simulink model "ADCS_FP5_RJF_Linear"  (R2024b)
settings: Solver=VariableStepAuto  StartTime=0.0  StopTime=tspan  FixedStep=10  RelTol=1e-4
values from neighbouring files (symbols this model uses):
  E_b_ECI_0 = rotm2eul(C_b_ECI_0)    [AERO421_FP5_RJF.m]
  J = diag([1200,2000,2800])    [AERO421_FP5_RJF.m]
  K = -15    [AERO421_FP5_RJF.m]
  q_b_ECI_0 = -rotm2quat(C_b_ECI_0)    [AERO421_FP5_RJF.m]
  T = [0;0;0]    [AERO421_FP5_RJF.m]
  w_b_ECI_0 = [-0.05; 0.03; 0.2]    [AERO421_FP5_RJF.m]
undefined symbols (not defined in the file or in its folder): Kd, Kp
settings Model: Creator=emehiel  LastModifiedBy=rosha
settings SolverCC: AlgebraicLoopSolver=TrustRegion
settings DebuggingCC: UnconnectedInputMsg=warning  UnconnectedOutputMsg=warning  UnconnectedLineMsg=warning
settings ModelReferenceCC: EnableRefExpFcnMdlSchedulingChecks=on
settings RTWCC: GPUComputeCapability=3.5

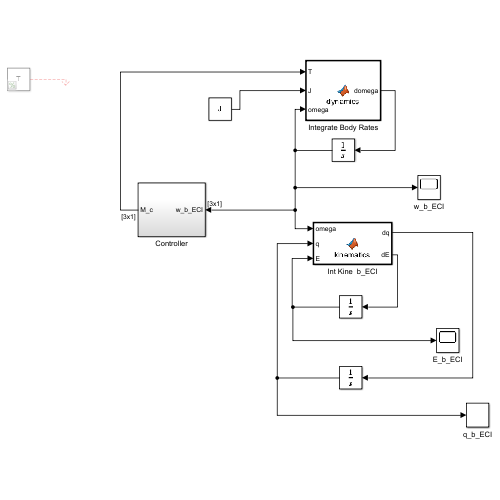
[thumbnail: Simulink's stored preview of the top-level diagram]
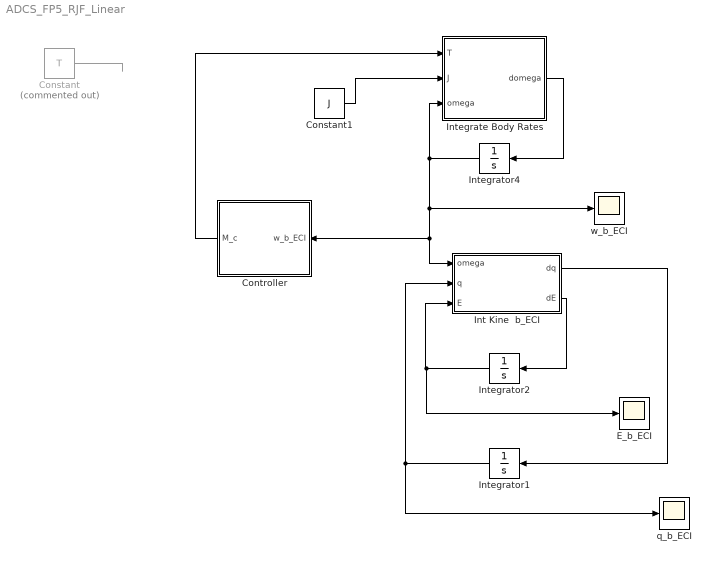
== system ADCS_FP5_RJF_Linear ==
  Constant : Constant  Commented=on  Value=T
  Constant1 : Constant  Value=J
  Controller : Subsystem
  E_b_ECI : Scope
  Int Kine  b_ECI : MATLAB Function  TreatAsAtomicUnit=on
  Integrate Body Rates : MATLAB Function  TreatAsAtomicUnit=on
  Integrator1 : Integrator  InitialCondition=q_b_ECI_0
  Integrator2 : Integrator  InitialCondition=E_b_ECI_0
  Integrator4 : Integrator  InitialCondition=w_b_ECI_0
  q_b_ECI : Scope
  w_b_ECI : Scope
  wires:
  Constant/1 -> ?
  Constant1/1 -> Integrate Body Rates/2(J)
  Integrate Body Rates/1(domega) -> Integrator4/1
  Integrator4/1 -> Controller/1(w_b_ECI), Int Kine  b_ECI/1(omega), w_b_ECI/1, Integrate Body Rates/3(omega)
  Integrator2/1 -> E_b_ECI/1, Int Kine  b_ECI/3(E)
  Int Kine  b_ECI/2(dE) -> Integrator2/1
  Int Kine  b_ECI/1(dq) -> Integrator1/1
  Controller/1(M_c) -> Integrate Body Rates/1(T)
  Integrator1/1 -> q_b_ECI/1, Int Kine  b_ECI/2(q)

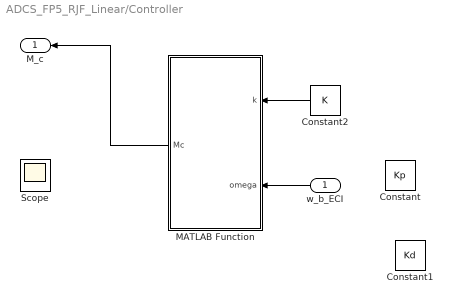
== system ADCS_FP5_RJF_Linear/Controller ==
  w_b_ECI : Inport  PortDimensions=[3 1]
  Constant : Constant  Value=Kp
  Constant1 : Constant  Value=Kd
  Constant2 : Constant  Value=K
  MATLAB Function : MATLAB Function  TreatAsAtomicUnit=on
  Scope : Scope
  M_c : Outport  PortDimensions=[3 1]  VectorParamsAs1DForOutWhenUnconnected=off
  wires:
  MATLAB Function/1(Mc) -> M_c/1
  w_b_ECI/1 -> MATLAB Function/2(omega)
  Constant2/1 -> MATLAB Function/1(k)

== matlab function ADCS_FP5_RJF_Linear/Int Kine  b_ECI ==
  data: omega input; q input; dq output; E input; dE output
function [dq,dE] = kinematics(omega, q, E)
%#codegen

% unpack quaternion

epsilon = q(1:3,1);
eta = q(4,1);

depsilon = 1/2*(eta*eye(3) + vcross(epsilon))*omega;
deta = -1/2*epsilon'*omega;

dq = [depsilon; deta];

LBI = 1/cos(E(2))*[cos(E(2)) sin(E(1))*sin(E(2))  cos(E(1))*sin(E(2));
                   0         cos(E(1))*cos(E(2)) -sin(E(1))*cos(E(2));
                   0         sin(E(1))            cos(E(1))];

dE = LBI*omega;

== matlab function ADCS_FP5_RJF_Linear/Integrate Body Rates ==
  data: T input; J input; omega input; domega output
function domega = dynamics(T, J, omega)
%#codegen

domega = J\(T - cross(omega, J*omega));

== matlab function ADCS_FP5_RJF_Linear/Controller/MATLAB Function ==
  data: k input; Mc output; omega input
function Mc   = control_law(k, omega)
%#codegen

Mc = k*omega;
